simulink model "motorA"  (R2018b)
settings: Solver=VariableStepAuto  StartTime=0.0  StopTime=10.0  RelTol=1e-3
libraries: fl_lib x5, elec_lib x3, nesl_utility x3
settings Model: Creator=Prathamesh  LastModifiedBy=Prathamesh

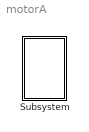
== system motorA ==
  Subsystem : Subsystem

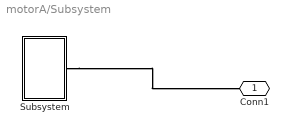
== system motorA/Subsystem ==
  Subsystem : Subsystem
  Conn1 : PMIOPort  Side=Right
  connections:
  Subsystem/RConn1 -- Conn1/RConn1

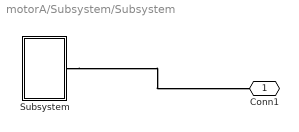
== system motorA/Subsystem/Subsystem ==
  Subsystem : Subsystem
  Conn1 : PMIOPort  Side=Right
  connections:
  Subsystem/RConn1 -- Conn1/RConn1

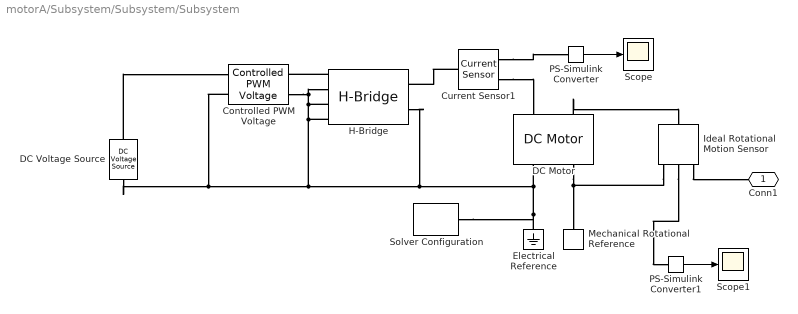
== system motorA/Subsystem/Subsystem/Subsystem ==
  Controlled PWM Voltage : elec_lib/Actuators & Drivers/Drivers/Controlled PWM Voltage  F=255 Hz  TD=0 s  pulse_width_offset=0 s  pulse_min=0 s  Vmin=0 V  Vmax=5 V  Vm=5 V  pwm_or_av=1  event_type=1  sample_time=1e-6 s  u_min=0  u_max=1
      settings: SourceProductName=Simscape Electronics  SourceProductBaseCode=SN
  Current Sensor1 : fl_lib/Electrical/Electrical Sensors/Current Sensor
  DC Motor : elec_lib/Actuators & Drivers/Rotational Actuators/DC Motor  parameterization=1  Ra=3.9 Ohm  La=12e-6 H  emf_or_torque=1  Kv=0.072e-3 V/rpm  Ki=6.876e-4 N*m/A  T_stall=0.24e-3 N*m  w_max=19100 rpm  w_rated=15000 rpm  P_rated=0.08 W  V_rated=1.5 V  J=0.01 g*cm^2  lam_param=1  lam=0 N*m/(rad/s)  i_noload=0 A  V_i_noload=1.5 V  speed0=0 rpm  alpha=3.93e-3 1/K  Tmeas=25 degC  thermal_mass=100 J/K  initial_temperature=25 degC
  DC Voltage Source : fl_lib/Electrical/Electrical Sources/DC Voltage Source  v0=12 V
  Electrical Reference : fl_lib/Electrical/Electrical Elements/Electrical Reference
  H-Bridge : elec_lib/Actuators & Drivers/Drivers/H-Bridge  Venable=2.5 V  Vmax=5.0 V  Vreverse=2.5 V  Vbrake=2.5 V  Vm=12 V  pwm_or_av=1  discontinuous=0  freewheeling_mode=1  freewheeling_mode_disc=1  Ron=0.1 Ohm  Don=0.05 Ohm  Rload=10 Ohm  Lload=1e-5 H  F=10 kHz  thermal_mass=100 J/K  initial_temperature=298.15 K  Ron2=0.1 Ohm  Don2=0.05 Ohm  Tmeas=298.15 K  Tmeas2=398.15 K
      settings: SourceProductName=Simscape Electronics  SourceProductBaseCode=SN
  Ideal Rotational Motion Sensor : fl_lib/Mechanical/Mechanical Sensors/Ideal Rotational Motion Sensor  offset=0 deg
  Mechanical Rotational Reference : fl_lib/Mechanical/Rotational Elements/Mechanical Rotational Reference
  PS-Simulink Converter : nesl_utility/PS-Simulink Converter  PhysicalDomain=network_engine_domain  SubClassName=ps_output  LeftPortType=input  RightPortType=output  PseudoPeriodic=off  Frequencies=[]  Unit=1  AffineConversion=off
  PS-Simulink Converter1 : nesl_utility/PS-Simulink Converter  PhysicalDomain=network_engine_domain  SubClassName=ps_output  LeftPortType=input  RightPortType=output  PseudoPeriodic=off  Frequencies=[]  Unit=1  AffineConversion=off
  Scope : Scope
  Scope1 : Scope
  Solver Configuration : nesl_utility/Solver Configuration  PhysicalDomain=network_engine_domain  SubClassName=solver  LeftPortType=input  RightPortType=generic  Tones=[]  Harmonics=[]  SimulateNoise=off  Profile=off  UseLocalSampling=off  EnableSwitchedLinearOptims=on  FrequencyDomain=off  UseCCode=off  RelTol=0.001  AbsTol=1e-06  MinStep=1e-09  ToWorkspace=off  RevertToSquareIcSolve=off  NumHomotopyIterations=100  PhasorMode=off  PhasorModeNumHarmonics=1  DoDC=off  ResidualTolerance=1e-09  UseLocalSolver=off  LocalSolverChoice=NE_BACKWARD_EULER_ADVANCER  LocalSolverSampleTime=0.001  DoFixedCost=off  MaxNonlinIter=3  MaxModeIter=2  LinearAlgebra=auto  EquationFormulation=NE_TIME_EF  DelaysMemoryBudget=1024  AutomaticFiltering=on  FilteringTimeConstant=0.001  PartitionStorageMethod=AS_NEEDED  PartitionMemoryBudget=1024
  Conn1 : PMIOPort  Side=Right
  wires:
  PS-Simulink Converter1/1 -> Scope1/1
  PS-Simulink Converter/1 -> Scope/1
  connections:
  Electrical Reference/LConn1 -- Solver Configuration/RConn1 -- H-Bridge/RConn2 -- H-Bridge/LConn4 -- H-Bridge/LConn3 -- H-Bridge/LConn2 -- Controlled PWM Voltage/RConn2 -- Controlled PWM Voltage/LConn2 -- DC Voltage Source/RConn1 -- DC Motor/RConn1
  H-Bridge/LConn1 -- Controlled PWM Voltage/RConn1
  DC Motor/LConn2 -- Ideal Rotational Motion Sensor/LConn1
  Ideal Rotational Motion Sensor/RConn3 -- Conn1/RConn1
  Current Sensor1/RConn1 -- PS-Simulink Converter/LConn1
  Current Sensor1/RConn2 -- DC Motor/LConn1
  DC Motor/RConn2 -- Ideal Rotational Motion Sensor/RConn1 -- Mechanical Rotational Reference/LConn1
  Current Sensor1/LConn1 -- H-Bridge/RConn1
  Ideal Rotational Motion Sensor/RConn2 -- PS-Simulink Converter1/LConn1
  DC Voltage Source/LConn1 -- Controlled PWM Voltage/LConn1
